simulink model "Rectificador_5_1_2026_optimizado"  (R2024a)
settings: Solver=VariableStepAuto  StartTime=0.0  StopTime=50  RelTol=1e-3
undefined symbols (not defined in the file): D1, Delta, DiscIntNeverNeededParam
libraries: spsSeriesRLCBranchLib x29, spsGroundLib x8, spsabctodq0Lib x4, simulink x4, spsUniversalBridgeLib x3, spsThreePhaseVIMeasurementLib x3, spsRMSLib x2, spsPWMGenerator2LevelLib x2, spsVoltageMeasurementLib x1, spsPower3phInstantaneousLib x1, spsPermanentMagnetSynchronousMachineLib x1, spsThreePhaseSourceLib x1
settings Model: PacingRate=1000  Creator=User  LastModifiedBy=User

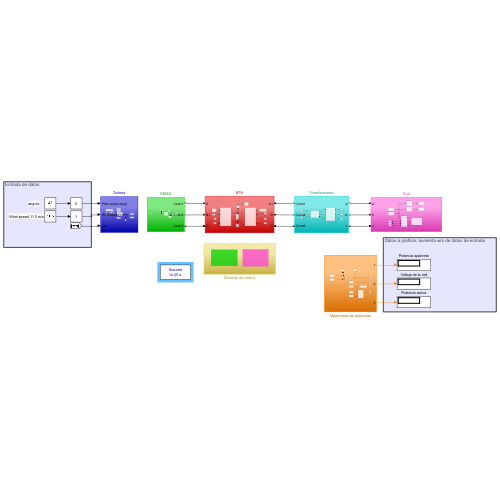
[thumbnail: Simulink's stored preview of the top-level diagram]
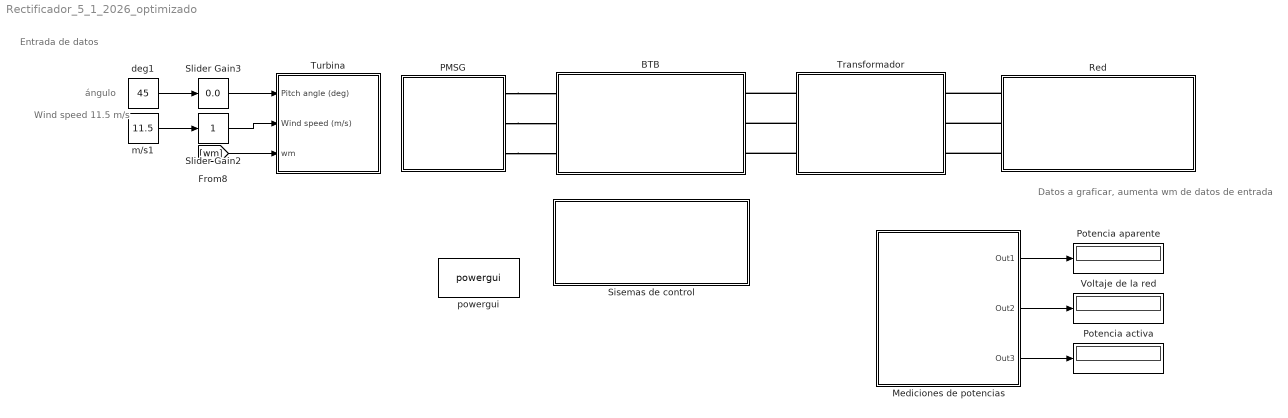
== system Rectificador_5_1_2026_optimizado ==
  note: Datos a graficar, aumenta wm de datos de entrada
  note: Wind speed 11.5 m/s
  note: ángulo
  note: Entrada de datos
  BTB : Subsystem
  Mediciones de potencias : Subsystem
  PMSG : Subsystem
  Potencia activa : Display
  Potencia aparente : Display
  Red : Subsystem
  Sisemas de control : Subsystem
  Slider Gain2 : simulink/Math Operations/Slider Gain  gain=1  low=0.2  high=1.0434782609
  Slider Gain3 : simulink/Math Operations/Slider Gain  gain=0.0  low=0  high=1
  Transformador : Subsystem
  Turbina : Subsystem
  Voltaje de la red : Display
  deg1 : Constant  Value=45  SampleTime=1e-6
  m/s1 : Constant  Value=11.5  SampleTime=1e-6
  powergui : spspowerguiLib/powergui  Priority=1  SimulationMode=Discrete  SampleTime=1e-5  frequency=60  Iterations=50  frequencyindice=0  Pbase=100e6  ErrMax=1e-4  UnitsV=kV  UnitsW=MW  buscounter=0  FunctionMessages=off  echomessages=off  EnableUseOfTLC=off  CurrentSourceSwitches=off  DisableSnubberDevices=off  DisableRonSwitches=off  DisableVfSwitches=off  DisplayEquations=off  AutomaticDiscreteSolvers=off  SolverType=Tustin/Backward Euler (TBE)  Interpol=off  ExternalGateDelay=off  methode=off  Ts=100  x0status=blocks  SPID=on  SwTol=0  HookPort=off  NonlinearTolerance=1e-4  nMaxIteration=100  ContinueOnMaxIteration=off  RestoreLinks=warning  ResistiveCurrentMeasurement=off  Frange=[0:2:500]  Ylog=off  Xlog=on  ShowGrid=off  save=off  variable=ZData  structure=0  ZoomFFT=off  StartTime=0.0  cycles=1  DisplayStyle=1  fundamental=60  FreqAxis=off  MaxFrequency=1000  frequencyindicesteady=1  RmsSteady=1  display=off
  wires:
  Slider Gain3/1 -> Turbina/1(Pitch angle (deg))
  deg1/1 -> Slider Gain3/1
  Slider Gain2/1 -> Turbina/2(Wind speed (m/s))
  m/s1/1 -> Slider Gain2/1
  [wm] -> Turbina/3(wm)
  Mediciones de potencias/1(Out1) -> Potencia aparente/1
  Mediciones de potencias/2(Out2) -> Voltaje de la red/1
  Mediciones de potencias/3(Out3) -> Potencia activa/1
  connections:
  PMSG/LConn1 -- BTB/RConn1
  PMSG/LConn2 -- BTB/RConn2
  PMSG/LConn3 -- BTB/RConn3
  Transformador/RConn1 -- BTB/LConn1
  Transformador/RConn2 -- BTB/LConn2
  Transformador/RConn3 -- BTB/LConn3
  Red/RConn1 -- Transformador/LConn1
  Red/RConn2 -- Transformador/LConn2
  Red/RConn3 -- Transformador/LConn3

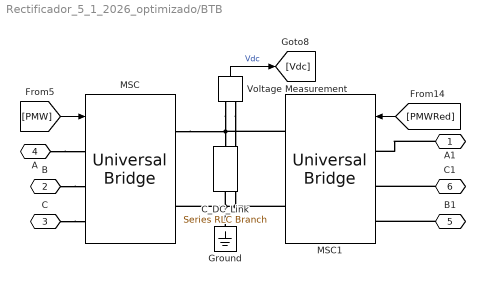
== system Rectificador_5_1_2026_optimizado/BTB ==
  C_DC_Link : spsSeriesRLCBranchLib/Series RLC Branch  LConnTagsString=__new0  RConnTagsString=__new0  BranchType=C  Resistance=1  Inductance=1e-3  SetiL0=off  InitialCurrent=0  Capacitance=5000e-6  Setx0=on  InitialVoltage=0  Measurements=None
  Ground : spsGroundLib/Ground  LConnTagsString=a
  MSC : spsUniversalBridgeLib/Universal Bridge  Arms=3  SnubberResistance=1e5  SnubberCapacitance=inf  Device=IGBT / Diodes  Ron=1e-3  Lon=0  ForwardVoltages=[ 0.8 , 0.8 ]  ForwardVoltage=0  GTOparameters=[ 10e-6 , 20e-6 ]  IGBTparameters=[ 1e-6 , 2e-6 ]  Measurements=None  Measurements_2=None  converterType=Rectifier
  MSC1 : spsUniversalBridgeLib/Universal Bridge  Arms=3  SnubberResistance=1e5  SnubberCapacitance=inf  Device=IGBT / Diodes  Ron=1e-3  Lon=0  ForwardVoltages=[ 0.8 , 0.8 ]  ForwardVoltage=0  GTOparameters=[ 10e-6 , 20e-6 ]  IGBTparameters=[ 1e-6 , 2e-6 ]  Measurements=None  Measurements_2=None  converterType=Rectifier
  Voltage Measurement : spsVoltageMeasurementLib/Voltage Measurement  PhasorSimulation=off  OutputType=Complex  PSBequivalent=0
  A1 : PMIOPort  Side=Left
  B : PMIOPort  Port=2  Side=Left
  C : PMIOPort  Port=3  Side=Left
  A : PMIOPort  Port=4  Side=Right
  B1 : PMIOPort  Port=5  Side=Right
  C1 : PMIOPort  Port=6  Side=Right
  wires:
  Voltage Measurement/1 -> [Vdc]  "Vdc"
  [PMWRed] -> MSC1/1
  [PMW] -> MSC/1
  connections:
  Voltage Measurement/LConn1 -- MSC1/RConn1 -- MSC/RConn1 -- C_DC_Link/LConn1
  A1/RConn1 -- MSC1/LConn1
  Voltage Measurement/LConn2 -- MSC/RConn2 -- Ground/LConn1 -- C_DC_Link/RConn1 -- MSC1/RConn2
  A/RConn1 -- MSC/LConn1
  B/RConn1 -- MSC/LConn2
  C/RConn1 -- MSC/LConn3
  C1/RConn1 -- MSC1/LConn2
  B1/RConn1 -- MSC1/LConn3

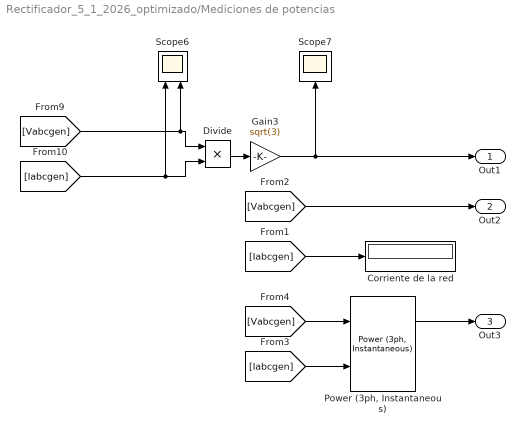
== system Rectificador_5_1_2026_optimizado/Mediciones de potencias ==
  Corriente de la red : Display
  Divide : Product  Inputs=**
  Gain3 : Gain  Gain=sqrt(3)
  "Power (3ph, Instantaneous)" : spsPower3phInstantaneousLib/Power (3ph, Instantaneous)
  Scope6 : Scope  NumInputPorts=2
  Scope7 : Scope
  Out1 : Outport
  Out2 : Outport  Port=2
  Out3 : Outport  Port=3
  wires:
  [Iabcgen] -> Divide/2, Scope6/2
  Gain3/1 -> Out1/1, Scope7/1
  [Iabcgen] -> Corriente de la red/1
  Divide/1 -> Gain3/1
  [Vabcgen] -> Scope6/1, Divide/1
  [Vabcgen] -> Out2/1
  [Vabcgen] -> "Power (3ph, Instantaneous)"/1
  [Iabcgen] -> "Power (3ph, Instantaneous)"/2
  "Power (3ph, Instantaneous)"/1 -> Out3/1

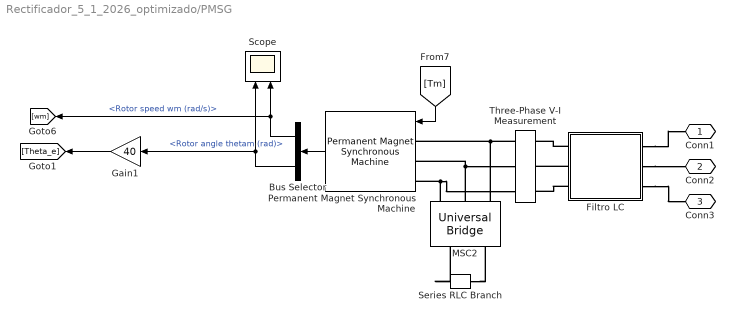
== system Rectificador_5_1_2026_optimizado/PMSG ==
  Bus Selector : BusSelector  OutputSignals=Rotor speed wm (rad/s),Rotor angle thetam (rad)
  Filtro LC : Subsystem
  Gain1 : Gain  Gain=40
  MSC2 : spsUniversalBridgeLib/Universal Bridge  Arms=3  SnubberResistance=1e5  SnubberCapacitance=inf  Device=Diodes  Ron=1e-3  Lon=0  ForwardVoltages=[ 0.8 , 0.8 ]  ForwardVoltage=0  GTOparameters=[ 10e-6 , 20e-6 ]  IGBTparameters=[ 1e-6 , 2e-6 ]  Measurements=None  Measurements_2=None  converterType=Rectifier
  Permanent Magnet Synchronous Machine : spsPermanentMagnetSynchronousMachineLib/Permanent Magnet Synchronous Machine  NbPhases=3  FluxDistribution=Sinusoidal  RotorType=Round  MechanicalLoad=Torque Tm  PresetModel=No  ShowDetailedParameters=on  MeasurementBus=off  Resistance=0.004  Inductance=8.5e-3  dqInductances=[8.5e-3,8.5e-3]  La=0.00175  MachineConstant=Flux linkage established by magnets (V.s)  Flux=5.85787  VoltageCst=42500.0035  TorqueCst=351.4722  Flat=120  Mechanical=[4e+06 1000 40]  PolePairs=4  InitialConditions=[0,0, 0,0]  InitialConditions5ph=[0 0 0 0 0 0]  RefAngle=90 degrees behind phase A axis (modified Park)  IterativeDiscreteModel=Trapezoidal non iterative  TsBlock=1e-06  TsPowergui=0
  Scope : Scope  NumInputPorts=2
  Series RLC Branch : spsSeriesRLCBranchLib/Series RLC Branch  LConnTagsString=__new0  RConnTagsString=__new0  BranchType=R  Resistance=100000  Inductance=1e-3  SetiL0=off  InitialCurrent=0  Capacitance=1e-6  Setx0=off  InitialVoltage=0  Measurements=None
  Three-Phase V-I Measurement : spsThreePhaseVIMeasurementLib/Three-Phase V-I Measurement  VoltageMeasurement=phase-to-ground  SetLabelV=on  LabelV=Vabc_gen  Vpu=off  VpuLL=off  CurrentMeasurement=yes  SetLabelI=on  LabelI=Iabc_gen  Ipu=off  Pbase=100e6  Vbase=500e3  OutputType=Complex  PhasorSimulation=off  PSBequivalent=0
  Conn1 : PMIOPort  Side=Left
  Conn2 : PMIOPort  Port=2  Side=Left
  Conn3 : PMIOPort  Port=3  Side=Left
  wires:
  Bus Selector/2 -> Gain1/1, Scope/2  "<Rotor angle thetam (rad)>"
  Gain1/1 -> [Theta_e]
  [Tm] -> Permanent Magnet Synchronous Machine/1
  Bus Selector/1 -> Scope/1, [wm]  "<Rotor speed wm (rad/s)>"
  Permanent Magnet Synchronous Machine/1 -> Bus Selector/1
  connections:
  Three-Phase V-I Measurement/RConn1 -- Permanent Magnet Synchronous Machine/LConn1 -- MSC2/LConn1
  MSC2/LConn2 -- Permanent Magnet Synchronous Machine/LConn2 -- Three-Phase V-I Measurement/RConn2
  MSC2/LConn3 -- Three-Phase V-I Measurement/RConn3 -- Permanent Magnet Synchronous Machine/LConn3
  Filtro LC/RConn3 -- Three-Phase V-I Measurement/LConn3
  Series RLC Branch/RConn1 -- MSC2/RConn2
  Filtro LC/RConn2 -- Three-Phase V-I Measurement/LConn2
  Series RLC Branch/LConn1 -- MSC2/RConn1
  Filtro LC/RConn1 -- Three-Phase V-I Measurement/LConn1
  Filtro LC/LConn2 -- Conn2/RConn1
  Filtro LC/LConn3 -- Conn3/RConn1
  Filtro LC/LConn1 -- Conn1/RConn1

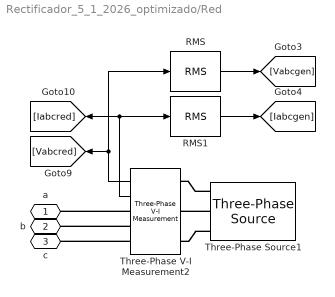
== system Rectificador_5_1_2026_optimizado/Red ==
  RMS : spsRMSLib/RMS  TrueRMS=on  Freq=60  RMSInit=120  Ts=1e-6
  RMS1 : spsRMSLib/RMS  TrueRMS=on  Freq=60  RMSInit=120  Ts=1e-6
  Three-Phase V-I Measurement2 : spsThreePhaseVIMeasurementLib/Three-Phase V-I Measurement  VoltageMeasurement=phase-to-phase  SetLabelV=off  LabelV=Vabc  Vpu=off  VpuLL=off  CurrentMeasurement=yes  SetLabelI=off  LabelI=Iabc  Ipu=off  Pbase=100e6  Vbase=500e3  OutputType=Complex  PhasorSimulation=off  PSBequivalent=0
  Three-Phase Source1 : spsThreePhaseSourceLib/Three-Phase Source  InternalConnection=Yg  VoltagePhases=off  Voltage=34.5e3  PhaseAngle=0  Voltage_phases=[25e3 25e3 25e3]/sqrt(3)  PhaseAngles_phases=[0 -120 +120]  Frequency=60  NonIdealSource=on  SpecifyImpedance=off  Resistance=1e-12  Inductance=1e-12  ShortCircuitLevel=100e6  BaseVoltage=34.5e3  XRratio=7  BusType=swing  Pref=10e3  Qref=0  Prefabc=[10e3, 10e3, 10e3]  Qrefabc=[0, 0, 0]  Qmin=-inf  Qmax=inf
  a : PMIOPort  Side=Right
  b : PMIOPort  Port=2  Side=Right
  c : PMIOPort  Port=3  Side=Right
  wires:
  Three-Phase V-I Measurement2/1 -> [Vabcred], RMS/1
  RMS/1 -> [Vabcgen]
  Three-Phase V-I Measurement2/2 -> [Iabcred], RMS1/1
  RMS1/1 -> [Iabcgen]
  connections:
  Three-Phase Source1/RConn2 -- Three-Phase V-I Measurement2/LConn2
  Three-Phase Source1/RConn1 -- Three-Phase V-I Measurement2/LConn1
  Three-Phase V-I Measurement2/RConn2 -- b/RConn1
  Three-Phase Source1/RConn3 -- Three-Phase V-I Measurement2/LConn3
  Three-Phase V-I Measurement2/RConn3 -- c/RConn1
  Three-Phase V-I Measurement2/RConn1 -- a/RConn1

== system Rectificador_5_1_2026_optimizado/Sisemas de control ==
  Sistema control lado de la red : Subsystem
  Sistema de control lado de PMSG : Subsystem

== system Rectificador_5_1_2026_optimizado/Transformador ==
  Filtro LCL : Subsystem
  Three-Phase Transformer (Two Windings) : spsThreePhaseTransformerTwoWindingsLib/Three-Phase Transformer (Two Windings)  Winding1Connection=Delta (D1)  Winding2Connection=Yg  CoreType=Three single-phase transformers  SetSaturation=off  Hysteresis=off  DataFile='hysteresis'  SetInitialFlux=off  Measurements=None  UNITS=SI  NominalPower=[ 4.4e6 , 60 ]  Winding1=[ 690 , 0.00558 , 1.92e-5]  Winding2=[ 34.5e3 ,1.395 , 0.00048]  Rm=1000  Lm=0.5  L0=0.5  Saturation=[0 0;0.66653 1910.3;277.72 2419.7]  InitialFluxes=[ 0.8 , -0.8 , 0.7 ]  BreakLoop=off  DiscreteSolver=Trapezoidal iterative  DataType=on  TransfoNumber=1
  a : PMIOPort  Side=Left
  b : PMIOPort  Port=2  Side=Left
  c : PMIOPort  Port=3  Side=Left
  Conn1 : PMIOPort  Port=4  Side=Right
  Conn4 : PMIOPort  Port=5  Side=Right
  Conn6 : PMIOPort  Port=6  Side=Right
  connections:
  Filtro LCL/RConn2 -- Conn4/RConn1
  Three-Phase Transformer (Two Windings)/LConn3 -- Filtro LCL/LConn3
  Three-Phase Transformer (Two Windings)/LConn2 -- Filtro LCL/LConn2
  a/RConn1 -- Three-Phase Transformer (Two Windings)/RConn1
  c/RConn1 -- Three-Phase Transformer (Two Windings)/RConn3
  Three-Phase Transformer (Two Windings)/LConn1 -- Filtro LCL/LConn1
  Filtro LCL/RConn1 -- Conn1/RConn1
  b/RConn1 -- Three-Phase Transformer (Two Windings)/RConn2
  Filtro LCL/RConn3 -- Conn6/RConn1

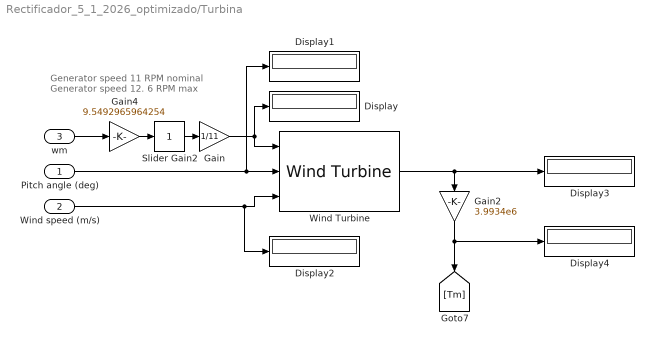
== system Rectificador_5_1_2026_optimizado/Turbina ==
  note: Generator speed 11 RPM nominal
      | Generator speed 12. 6 RPM max
  Pitch angle (deg) : Inport
  Wind speed (m/s) : Inport  Port=2
  wm : Inport  Port=3
  Display{,1..4} (5 alike) : Display
  Gain : Gain  Gain=1/11
  Gain2 : Gain  Gain=3.9934e6
  Gain4 : Gain  Gain=9.5492965964254
  Slider Gain2 : simulink/Math Operations/Slider Gain  gain=1  low=0.2  high=1.145
  Wind Turbine : spsWindTurbineLib/Wind Turbine  Pnom=4.59e6  Pelec_base=4.59e6  wind_base=11.5  P_wind_base=1  speed_nom=1  pitch_angle=0  c1_c6="[0.51763          116          0.4            5           21     0.006795]"  cp_nom=0.48  lambda_nom=8.1
  wires:
  Gain/1 -> Wind Turbine/1, Display/1
  Wind Turbine/1 -> Display3/1, Gain2/1
  Gain4/1 -> Slider Gain2/1
  wm/1 -> Gain4/1
  Gain2/1 -> [Tm], Display4/1
  Pitch angle (deg)/1 -> Display1/1, Wind Turbine/2
  Slider Gain2/1 -> Gain/1
  Wind speed (m/s)/1 -> Wind Turbine/3, Display2/1

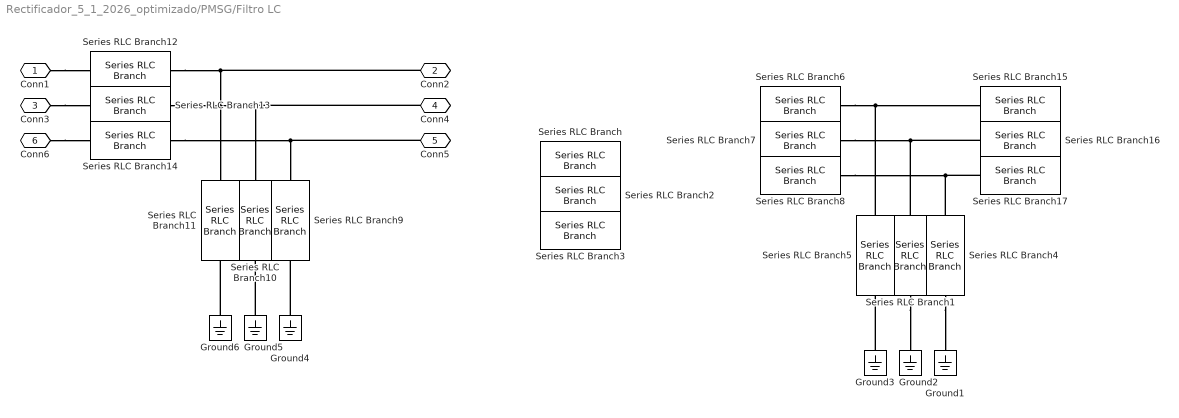
== system Rectificador_5_1_2026_optimizado/PMSG/Filtro LC ==
  Ground{1..6} (6 alike) : spsGroundLib/Ground  LConnTagsString=a
  Series RLC Branch : spsSeriesRLCBranchLib/Series RLC Branch  LConnTagsString=__new0  RConnTagsString=__new0  BranchType=L  Resistance=1  Inductance=8.1685e-06  SetiL0=off  InitialCurrent=0  Capacitance=1e-6  Setx0=off  InitialVoltage=0  Measurements=None
  Series RLC Branch1 : spsSeriesRLCBranchLib/Series RLC Branch  LConnTagsString=__new0  RConnTagsString=__new0  BranchType=RC  Resistance=0  Inductance=1e-3  SetiL0=off  InitialCurrent=0  Capacitance=200e-6  Setx0=off  InitialVoltage=0  Measurements=None
  Series RLC Branch10 : spsSeriesRLCBranchLib/Series RLC Branch  LConnTagsString=__new0  RConnTagsString=__new0  BranchType=RC  Resistance=0.04  Inductance=1e-3  SetiL0=off  InitialCurrent=0  Capacitance=100e-06  Setx0=off  InitialVoltage=0  Measurements=None
  Series RLC Branch11 : spsSeriesRLCBranchLib/Series RLC Branch  LConnTagsString=__new0  RConnTagsString=__new0  BranchType=RC  Resistance=0.04  Inductance=1e-3  SetiL0=off  InitialCurrent=0  Capacitance=100e-06  Setx0=off  InitialVoltage=0  Measurements=None
  Series RLC Branch12 : spsSeriesRLCBranchLib/Series RLC Branch  LConnTagsString=__new0  RConnTagsString=__new0  BranchType=L  Resistance=1  Inductance=50e-04  SetiL0=off  InitialCurrent=0  Capacitance=1e-6  Setx0=off  InitialVoltage=0  Measurements=None
  Series RLC Branch13 : spsSeriesRLCBranchLib/Series RLC Branch  LConnTagsString=__new0  RConnTagsString=__new0  BranchType=L  Resistance=1  Inductance=50e-04  SetiL0=off  InitialCurrent=0  Capacitance=1e-6  Setx0=off  InitialVoltage=0  Measurements=None
  Series RLC Branch14 : spsSeriesRLCBranchLib/Series RLC Branch  LConnTagsString=__new0  RConnTagsString=__new0  BranchType=L  Resistance=1  Inductance=50e-04  SetiL0=off  InitialCurrent=0  Capacitance=1e-6  Setx0=off  InitialVoltage=0  Measurements=None
  Series RLC Branch15 : spsSeriesRLCBranchLib/Series RLC Branch  LConnTagsString=__new0  RConnTagsString=__new0  BranchType=L  Resistance=0  Inductance=0.1e-3  SetiL0=off  InitialCurrent=0  Capacitance=1e-6  Setx0=off  InitialVoltage=0  Measurements=None
  Series RLC Branch16 : spsSeriesRLCBranchLib/Series RLC Branch  LConnTagsString=__new0  RConnTagsString=__new0  BranchType=L  Resistance=0  Inductance=0.1e-3  SetiL0=off  InitialCurrent=0  Capacitance=1e-6  Setx0=off  InitialVoltage=0  Measurements=None
  Series RLC Branch17 : spsSeriesRLCBranchLib/Series RLC Branch  LConnTagsString=__new0  RConnTagsString=__new0  BranchType=L  Resistance=0  Inductance=0.1e-3  SetiL0=off  InitialCurrent=0  Capacitance=1e-6  Setx0=off  InitialVoltage=0  Measurements=None
  Series RLC Branch2 : spsSeriesRLCBranchLib/Series RLC Branch  LConnTagsString=__new0  RConnTagsString=__new0  BranchType=L  Resistance=1  Inductance=8.1685e-06  SetiL0=off  InitialCurrent=0  Capacitance=1e-6  Setx0=off  InitialVoltage=0  Measurements=None
  Series RLC Branch3 : spsSeriesRLCBranchLib/Series RLC Branch  LConnTagsString=__new0  RConnTagsString=__new0  BranchType=L  Resistance=1  Inductance=8.1685e-06  SetiL0=off  InitialCurrent=0  Capacitance=1e-6  Setx0=off  InitialVoltage=0  Measurements=None
  Series RLC Branch4 : spsSeriesRLCBranchLib/Series RLC Branch  LConnTagsString=__new0  RConnTagsString=__new0  BranchType=RC  Resistance=0  Inductance=1e-3  SetiL0=off  InitialCurrent=0  Capacitance=200e-6  Setx0=off  InitialVoltage=0  Measurements=None
  Series RLC Branch5 : spsSeriesRLCBranchLib/Series RLC Branch  LConnTagsString=__new0  RConnTagsString=__new0  BranchType=RC  Resistance=0  Inductance=1e-3  SetiL0=off  InitialCurrent=0  Capacitance=200e-6  Setx0=off  InitialVoltage=0  Measurements=None
  Series RLC Branch6 : spsSeriesRLCBranchLib/Series RLC Branch  LConnTagsString=__new0  RConnTagsString=__new0  BranchType=L  Resistance=0  Inductance=3e-3  SetiL0=off  InitialCurrent=0  Capacitance=1e-6  Setx0=off  InitialVoltage=0  Measurements=None
  Series RLC Branch7 : spsSeriesRLCBranchLib/Series RLC Branch  LConnTagsString=__new0  RConnTagsString=__new0  BranchType=L  Resistance=0  Inductance=3e-3  SetiL0=off  InitialCurrent=0  Capacitance=1e-6  Setx0=off  InitialVoltage=0  Measurements=None
  Series RLC Branch8 : spsSeriesRLCBranchLib/Series RLC Branch  LConnTagsString=__new0  RConnTagsString=__new0  BranchType=L  Resistance=0  Inductance=3e-3  SetiL0=off  InitialCurrent=0  Capacitance=1e-6  Setx0=off  InitialVoltage=0  Measurements=None
  Series RLC Branch9 : spsSeriesRLCBranchLib/Series RLC Branch  LConnTagsString=__new0  RConnTagsString=__new0  BranchType=RC  Resistance=0.04  Inductance=1e-3  SetiL0=off  InitialCurrent=0  Capacitance=100e-06  Setx0=off  InitialVoltage=0  Measurements=None
  Conn1 : PMIOPort  Side=Left
  Conn2 : PMIOPort  Port=2  Side=Right
  Conn3 : PMIOPort  Port=3  Side=Left
  Conn4 : PMIOPort  Port=4  Side=Right
  Conn5 : PMIOPort  Port=5  Side=Right
  Conn6 : PMIOPort  Port=6  Side=Left
  connections:
  Series RLC Branch4/RConn1 -- Ground1/LConn1
  Series RLC Branch1/RConn1 -- Ground2/LConn1
  Ground3/LConn1 -- Series RLC Branch5/RConn1
  Series RLC Branch6/RConn1 -- Series RLC Branch5/LConn1 -- Series RLC Branch15/LConn1
  Series RLC Branch7/RConn1 -- Series RLC Branch1/LConn1 -- Series RLC Branch16/LConn1
  Series RLC Branch8/RConn1 -- Series RLC Branch4/LConn1 -- Series RLC Branch17/LConn1
  Series RLC Branch13/RConn1 -- Conn4/RConn1 -- Series RLC Branch10/LConn1
  Series RLC Branch12/RConn1 -- Conn2/RConn1 -- Series RLC Branch11/LConn1
  Series RLC Branch14/RConn1 -- Conn5/RConn1 -- Series RLC Branch9/LConn1
  Ground6/LConn1 -- Series RLC Branch11/RConn1
  Ground4/LConn1 -- Series RLC Branch9/RConn1
  Ground5/LConn1 -- Series RLC Branch10/RConn1
  Conn1/RConn1 -- Series RLC Branch12/LConn1
  Conn3/RConn1 -- Series RLC Branch13/LConn1
  Conn6/RConn1 -- Series RLC Branch14/LConn1

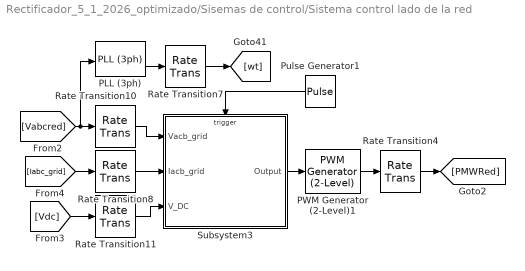
== system Rectificador_5_1_2026_optimizado/Sisemas de control/Sistema control lado de la red ==
  PLL (3ph) : spsPLL3phLib/PLL (3ph)  Fmin=45  Par_Init=[0, 60]  ParK=[180, 3200, 1]  TcD=1e-4  MaxRateChangeFreq=12  FilterCutOffFreq=25  Ts=0  AGC=on
  PWM Generator (2-Level)1 : spsPWMGenerator2LevelLib/PWM Generator (2-Level)  ModulatorType=Three-phase bridge (6 pulses)  ModulatorMode=Unsynchronized  Fc=10000  Pc=90  nF=27  MinMax="[ -1  1 ]"  SamplingTechnique=Natural  ModulatingSignals=off  m=0.8  Freq=60  Phase=0  Ts=1e-6  ShowCarrierOutport=off
  Pulse Generator1 : DiscretePulseGenerator  PulseType=Time based  Period=1e-3  PulseWidth=50
  Rate Transition{4,7..8,10..11} (5 alike) : RateTransition
  Subsystem3 : Subsystem
  wires:
  Rate Transition10/1 -> Subsystem3/1(Vacb_grid)
  [Vabcred] -> PLL (3ph)/1, Rate Transition10/1
  Subsystem3/1(Output) -> PWM Generator (2-Level)1/1
  Pulse Generator1/1 -> Subsystem3/Trigger
  Rate Transition7/1 -> [wt]
  Rate Transition11/1 -> Subsystem3/3(V_DC)
  [Iabc_grid] -> Rate Transition8/1
  [Vdc] -> Rate Transition11/1
  Rate Transition4/1 -> [PMWRed]
  Rate Transition8/1 -> Subsystem3/2(Iacb_grid)
  PLL (3ph)/2 -> Rate Transition7/1
  PWM Generator (2-Level)1/1 -> Rate Transition4/1

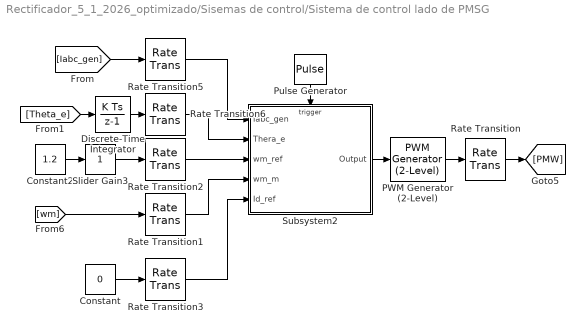
== system Rectificador_5_1_2026_optimizado/Sisemas de control/Sistema de control lado de PMSG ==
  Constant : Constant  Value=0  SampleTime=-1
  Constant2 : Constant  Value=1.2  SampleTime=-1
  Discrete-Time Integrator : DiscreteIntegrator  SampleTime=-1  ICPrevOutput=DiscIntNeverNeededParam  ICPrevScaledInput=DiscIntNeverNeededParam
  PWM Generator (2-Level) : spsPWMGenerator2LevelLib/PWM Generator (2-Level)  ModulatorType=Three-phase bridge (6 pulses)  ModulatorMode=Unsynchronized  Fc=10000  Pc=90  nF=27  MinMax="[ -1  1 ]"  SamplingTechnique=Natural  ModulatingSignals=off  m=0.8  Freq=60  Phase=0  Ts=1e-6  ShowCarrierOutport=off
  Pulse Generator : DiscretePulseGenerator  PulseType=Time based  Period=1e-3  PulseWidth=50
  Rate Transition{,1..3,5..6} (6 alike) : RateTransition
  Slider Gain3 : simulink/Math Operations/Slider Gain  gain=1  low=0.2  high=1.145
  Subsystem2 : Subsystem
  wires:
  PWM Generator (2-Level)/1 -> Rate Transition/1
  Pulse Generator/1 -> Subsystem2/Trigger
  Discrete-Time Integrator/1 -> Rate Transition6/1
  Subsystem2/1(Output) -> PWM Generator (2-Level)/1
  Rate Transition2/1 -> Subsystem2/3(wm_ref)
  Rate Transition5/1 -> Subsystem2/1(Iabc_gen)
  Rate Transition6/1 -> Subsystem2/2(Thera_e)
  [Iabc_gen] -> Rate Transition5/1
  Slider Gain3/1 -> Rate Transition2/1
  Rate Transition/1 -> [PMW]
  [Theta_e] -> Discrete-Time Integrator/1
  Constant/1 -> Rate Transition3/1
  Rate Transition1/1 -> Subsystem2/4(wm_m)
  [wm] -> Rate Transition1/1
  Rate Transition3/1 -> Subsystem2/5(Id_ref)
  Constant2/1 -> Slider Gain3/1

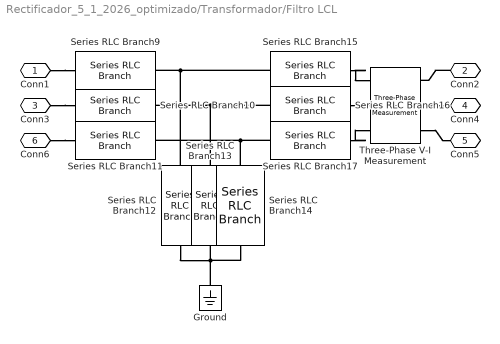
== system Rectificador_5_1_2026_optimizado/Transformador/Filtro LCL ==
  Ground : spsGroundLib/Ground  LConnTagsString=a
  Series RLC Branch10 : spsSeriesRLCBranchLib/Series RLC Branch  LConnTagsString=__new0  RConnTagsString=__new0  BranchType=RL  Resistance=0.07  Inductance=7.2924e-06  SetiL0=off  InitialCurrent=0  Capacitance=1e-6  Setx0=off  InitialVoltage=0  Measurements=None
  Series RLC Branch11 : spsSeriesRLCBranchLib/Series RLC Branch  LConnTagsString=__new0  RConnTagsString=__new0  BranchType=RL  Resistance=0.07  Inductance=7.2924e-06  SetiL0=off  InitialCurrent=0  Capacitance=1e-6  Setx0=off  InitialVoltage=0  Measurements=None
  Series RLC Branch12 : spsSeriesRLCBranchLib/Series RLC Branch  LConnTagsString=__new0  RConnTagsString=__new0  BranchType=RC  Resistance=0.002  Inductance=1e-3  SetiL0=off  InitialCurrent=0  Capacitance=4.3858e-04  Setx0=off  InitialVoltage=0  Measurements=None
  Series RLC Branch13 : spsSeriesRLCBranchLib/Series RLC Branch  LConnTagsString=__new0  RConnTagsString=__new0  BranchType=RC  Resistance=0.002  Inductance=1e-3  SetiL0=off  InitialCurrent=0  Capacitance=4.3858e-04  Setx0=off  InitialVoltage=0  Measurements=None
  Series RLC Branch14 : spsSeriesRLCBranchLib/Series RLC Branch  LConnTagsString=__new0  RConnTagsString=__new0  BranchType=RC  Resistance=0.002  Inductance=1e-3  SetiL0=off  InitialCurrent=0  Capacitance=4.3858e-04  Setx0=off  InitialVoltage=0  Measurements=None
  Series RLC Branch15 : spsSeriesRLCBranchLib/Series RLC Branch  LConnTagsString=__new0  RConnTagsString=__new0  BranchType=L  Resistance=1  Inductance=1.6043e-04  SetiL0=off  InitialCurrent=0  Capacitance=1e-6  Setx0=off  InitialVoltage=0  Measurements=None
  Series RLC Branch16 : spsSeriesRLCBranchLib/Series RLC Branch  LConnTagsString=__new0  RConnTagsString=__new0  BranchType=L  Resistance=1  Inductance=1.6043e-04  SetiL0=off  InitialCurrent=0  Capacitance=1e-6  Setx0=off  InitialVoltage=0  Measurements=None
  Series RLC Branch17 : spsSeriesRLCBranchLib/Series RLC Branch  LConnTagsString=__new0  RConnTagsString=__new0  BranchType=L  Resistance=1  Inductance=1.6043e-04  SetiL0=off  InitialCurrent=0  Capacitance=1e-6  Setx0=off  InitialVoltage=0  Measurements=None
  Series RLC Branch9 : spsSeriesRLCBranchLib/Series RLC Branch  LConnTagsString=__new0  RConnTagsString=__new0  BranchType=RL  Resistance=0.07  Inductance=7.2924e-06  SetiL0=off  InitialCurrent=0  Capacitance=1e-6  Setx0=off  InitialVoltage=0  Measurements=None
  Three-Phase V-I Measurement : spsThreePhaseVIMeasurementLib/Three-Phase V-I Measurement  VoltageMeasurement=no  SetLabelV=off  LabelV=Vabc  Vpu=off  VpuLL=off  CurrentMeasurement=yes  SetLabelI=on  LabelI=Iabc_grid  Ipu=off  Pbase=100e6  Vbase=500e3  OutputType=Complex  PhasorSimulation=off  PSBequivalent=0
  Conn1 : PMIOPort  Side=Left
  Conn2 : PMIOPort  Port=2  Side=Right
  Conn3 : PMIOPort  Port=3  Side=Left
  Conn4 : PMIOPort  Port=4  Side=Right
  Conn5 : PMIOPort  Port=5  Side=Right
  Conn6 : PMIOPort  Port=6  Side=Left
  connections:
  Series RLC Branch17/LConn1 -- Series RLC Branch14/LConn1 -- Series RLC Branch11/RConn1
  Series RLC Branch12/RConn1 -- Ground/LConn1 -- Series RLC Branch14/RConn1 -- Series RLC Branch13/RConn1
  Series RLC Branch15/LConn1 -- Series RLC Branch12/LConn1 -- Series RLC Branch9/RConn1
  Series RLC Branch16/LConn1 -- Series RLC Branch13/LConn1 -- Series RLC Branch10/RConn1
  Conn1/RConn1 -- Series RLC Branch9/LConn1
  Conn3/RConn1 -- Series RLC Branch10/LConn1
  Conn6/RConn1 -- Series RLC Branch11/LConn1
  Series RLC Branch15/RConn1 -- Three-Phase V-I Measurement/LConn1
  Series RLC Branch16/RConn1 -- Three-Phase V-I Measurement/LConn2
  Series RLC Branch17/RConn1 -- Three-Phase V-I Measurement/LConn3
  Three-Phase V-I Measurement/RConn2 -- Conn4/RConn1
  Conn2/RConn1 -- Three-Phase V-I Measurement/RConn1
  Three-Phase V-I Measurement/RConn3 -- Conn5/RConn1

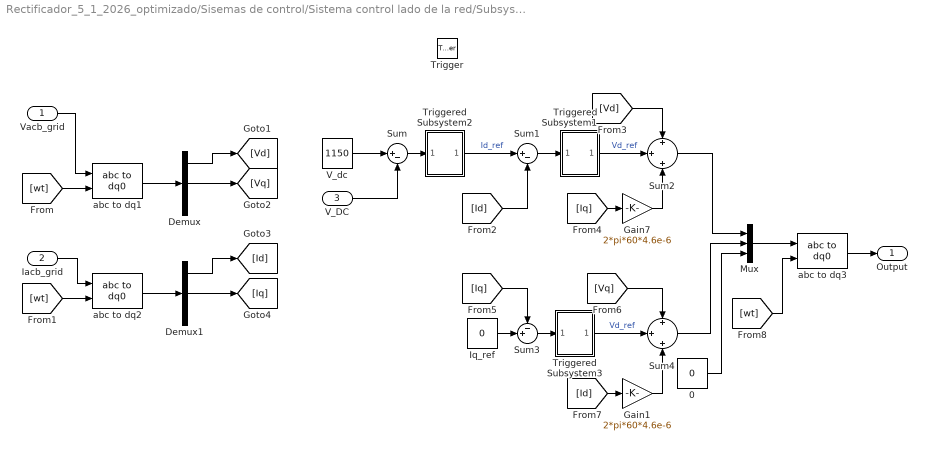
== system Rectificador_5_1_2026_optimizado/Sisemas de control/Sistema control lado de la red/Subsystem3 ==
  Vacb_grid : Inport
  Iacb_grid : Inport  Port=2
  V_DC : Inport  Port=3
  Trigger : TriggerPort  VariantControl=(inherit)
  0 : Constant  Value=0  SampleTime=-1
  Demux : Demux  Outputs=3
  Demux1 : Demux  Outputs=3
  Gain1 : Gain  Gain=2*pi*60*4.6e-6
  Gain7 : Gain  Gain=2*pi*60*4.6e-6
  Iq_ref : Constant  Value=0  SampleTime=-1
  Mux : Mux  Inputs=3
  Sum : Sum  Inputs=|+-
  Sum1 : Sum  Inputs=|+-
  Sum2 : Sum  Inputs=+|+|+
  Sum3 : Sum  Inputs=-+|
  Sum4 : Sum  Inputs=+|+|+
  Triggered Subsystem1 : Subsystem  TreatAsAtomicUnit=on
  Triggered Subsystem2 : Subsystem  TreatAsAtomicUnit=on
  Triggered Subsystem3 : Subsystem  TreatAsAtomicUnit=on
  V_dc : Constant  Value=1150  SampleTime=-1
  abc to dq1 : spsabctodq0Lib/abc to dq0  Alignment=90 degrees behind phase A axis
  abc to dq2 : spsabctodq0Lib/abc to dq0  Alignment=90 degrees behind phase A axis
  abc to dq3 : spsabctodq0Lib/abc to dq0  Alignment=90 degrees behind phase A axis
  Output : Outport
  wires:
  [wt] -> abc to dq1/2
  abc to dq1/1 -> Demux/1
  Demux/1 -> [Vd]
  Demux/2 -> [Vq]
  [wt] -> abc to dq2/2
  Iacb_grid/1 -> abc to dq2/1
  abc to dq2/1 -> Demux1/1
  Demux1/2 -> [Iq]
  Demux1/1 -> [Id]
  V_dc/1 -> Sum/1
  V_DC/1 -> Sum/2
  Sum/1 -> Triggered Subsystem2/1(In1)
  Vacb_grid/1 -> abc to dq1/1
  Triggered Subsystem2/1(Out1) -> Sum1/1  "Id_ref"
  [Id] -> Sum1/2
  Sum1/1 -> Triggered Subsystem1/1(In1)
  Triggered Subsystem1/1(Out1) -> Sum2/2  "Vd_ref"
  [Vd] -> Sum2/1
  [Iq] -> Gain7/1
  Gain7/1 -> Sum2/3
  Iq_ref/1 -> Sum3/2
  [Iq] -> Sum3/1
  Sum3/1 -> Triggered Subsystem3/1(In1)
  Triggered Subsystem3/1(Out1) -> Sum4/2  "Vd_ref"
  [Vq] -> Sum4/1
  [Id] -> Gain1/1
  Gain1/1 -> Sum4/3
  Sum2/1 -> Mux/1
  Sum4/1 -> Mux/2
  0/1 -> Mux/3
  Mux/1 -> abc to dq3/1
  [wt] -> abc to dq3/2
  abc to dq3/1 -> Output/1

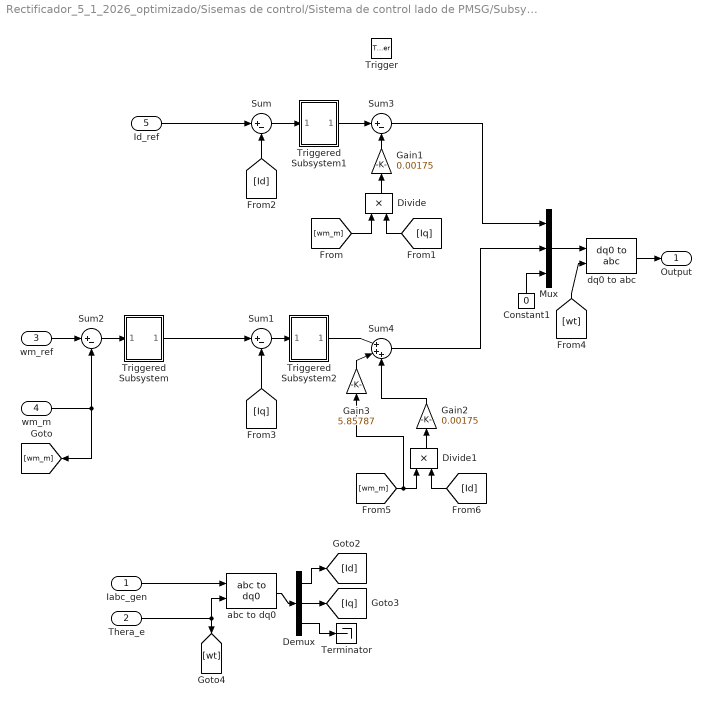
== system Rectificador_5_1_2026_optimizado/Sisemas de control/Sistema de control lado de PMSG/Subsystem2 ==
  Iabc_gen : Inport
  Thera_e : Inport  Port=2
  wm_ref : Inport  Port=3
  wm_m : Inport  Port=4
  Id_ref : Inport  Port=5
  Trigger : TriggerPort  VariantControl=(inherit)
  Constant1 : Constant  Value=0
  Demux : Demux  Outputs=3
  Divide : Product  Inputs=**
  Divide1 : Product  Inputs=**
  Gain1 : Gain  Gain=0.00175
  Gain2 : Gain  Gain=0.00175
  Gain3 : Gain  Gain=5.85787
  Mux : Mux  Inputs=3
  Sum{,1..3} (4 alike) : Sum  Inputs=|+-
  Sum4 : Sum  Inputs=|+++
  Terminator : Terminator
  Triggered Subsystem : Subsystem  TreatAsAtomicUnit=on
  Triggered Subsystem1 : Subsystem  TreatAsAtomicUnit=on
  Triggered Subsystem2 : Subsystem  TreatAsAtomicUnit=on
  abc to dq0 : spsabctodq0Lib/abc to dq0  Alignment=90 degrees behind phase A axis
  dq0 to abc : spsdq0toabcLib/dq0 to abc  Alignment=90 degrees behind phase A axis
  Output : Outport
  wires:
  [Id] -> Sum/2
  Sum/1 -> Triggered Subsystem1/1(In1)
  Sum2/1 -> Triggered Subsystem/1(In1)
  wm_ref/1 -> Sum2/1
  Demux/2 -> [Iq]
  Demux/1 -> [Id]
  [wt] -> dq0 to abc/2
  Sum1/1 -> Triggered Subsystem2/1(In1)
  [Iq] -> Sum1/2
  Mux/1 -> dq0 to abc/1
  abc to dq0/1 -> Demux/1
  Thera_e/1 -> [wt], abc to dq0/2
  Demux/3 -> Terminator/1
  Constant1/1 -> Mux/3
  dq0 to abc/1 -> Output/1
  Iabc_gen/1 -> abc to dq0/1
  wm_m/1 -> Sum2/2, [wm_m]
  Id_ref/1 -> Sum/1
  Triggered Subsystem1/1(Out1) -> Sum3/1
  Sum3/1 -> Mux/1
  Gain1/1 -> Sum3/2
  Divide/1 -> Gain1/1
  [Iq] -> Divide/2
  [wm_m] -> Divide/1
  Triggered Subsystem2/1(Out1) -> Sum4/1
  Gain2/1 -> Sum4/3
  Divide1/1 -> Gain2/1
  [wm_m] -> Gain3/1, Divide1/1
  [Id] -> Divide1/2
  Gain3/1 -> Sum4/2
  Sum4/1 -> Mux/2
  Triggered Subsystem/1(Out1) -> Sum1/1

== system Rectificador_5_1_2026_optimizado/Sisemas de control/Sistema control lado de la red/Subsystem3/Triggered Subsystem1 ==
  In1 : Inport
  Add : Sum
  Discrete-Time Integrator : DiscreteIntegrator  SampleTime=-1  IgnoreLimit=on  ICPrevOutput=DiscIntNeverNeededParam  ICPrevScaledInput=DiscIntNeverNeededParam
  Gain : Gain  Gain=0.0602
  Gain1 : Gain  Gain=5000
  Saturation : Saturate  UpperLimit=1150  LowerLimit=-1150
  Out1 : Outport
  wires:
  Gain1/1 -> Discrete-Time Integrator/1
  Discrete-Time Integrator/1 -> Add/2
  Gain/1 -> Add/1
  In1/1 -> Gain1/1, Gain/1
  Add/1 -> Out1/1

== system Rectificador_5_1_2026_optimizado/Sisemas de control/Sistema control lado de la red/Subsystem3/Triggered Subsystem2 ==
  In1 : Inport
  Add : Sum
  Discrete-Time Integrator : DiscreteIntegrator  SampleTime=-1  IgnoreLimit=on  ICPrevOutput=DiscIntNeverNeededParam  ICPrevScaledInput=DiscIntNeverNeededParam
  Gain : Gain  Gain=379.5
  Gain1 : Gain  Gain=0.031
  Saturation : Saturate  UpperLimit=1150  LowerLimit=-1150
  Out1 : Outport
  wires:
  Gain1/1 -> Discrete-Time Integrator/1
  Discrete-Time Integrator/1 -> Add/2
  Gain/1 -> Add/1
  In1/1 -> Gain1/1, Gain/1
  Add/1 -> Saturation/1
  Saturation/1 -> Out1/1

== system Rectificador_5_1_2026_optimizado/Sisemas de control/Sistema control lado de la red/Subsystem3/Triggered Subsystem3 ==
  In1 : Inport
  Add : Sum
  Discrete-Time Integrator : DiscreteIntegrator  SampleTime=-1  IgnoreLimit=on  ICPrevOutput=DiscIntNeverNeededParam  ICPrevScaledInput=DiscIntNeverNeededParam
  Gain : Gain  Gain=0.0602
  Gain1 : Gain  Gain=5000
  Saturation : Saturate  UpperLimit=1150  LowerLimit=-1150
  Out1 : Outport
  wires:
  Gain1/1 -> Discrete-Time Integrator/1
  Discrete-Time Integrator/1 -> Add/2
  Gain/1 -> Add/1
  In1/1 -> Gain1/1, Gain/1
  Add/1 -> Out1/1

== system Rectificador_5_1_2026_optimizado/Sisemas de control/Sistema de control lado de PMSG/Subsystem2/Triggered Subsystem ==
  In1 : Inport
  Add : Sum
  Discrete-Time Integrator : DiscreteIntegrator  SampleTime=-1  IgnoreLimit=on  ICPrevOutput=DiscIntNeverNeededParam  ICPrevScaledInput=DiscIntNeverNeededParam
  Gain : Gain
  Gain1 : Gain  Gain=50
  Saturation : Saturate  UpperLimit=4.5e6  LowerLimit=-4.5e6
  Out1 : Outport
  wires:
  Gain1/1 -> Discrete-Time Integrator/1
  Discrete-Time Integrator/1 -> Add/2
  Gain/1 -> Add/1
  In1/1 -> Gain1/1, Gain/1
  Add/1 -> Out1/1

== system Rectificador_5_1_2026_optimizado/Sisemas de control/Sistema de control lado de PMSG/Subsystem2/Triggered Subsystem1 ==
  In1 : Inport
  Add : Sum
  Discrete-Time Integrator : DiscreteIntegrator  SampleTime=-1  IgnoreLimit=on  ICPrevOutput=DiscIntNeverNeededParam  ICPrevScaledInput=DiscIntNeverNeededParam
  Gain : Gain  Gain=0.0602
  Gain1 : Gain  Gain=0.031
  Saturation : Saturate  UpperLimit=1150  LowerLimit=-1150
  Out1 : Outport
  wires:
  Gain1/1 -> Discrete-Time Integrator/1
  Discrete-Time Integrator/1 -> Add/2
  Gain/1 -> Add/1
  In1/1 -> Gain1/1, Gain/1
  Add/1 -> Out1/1

== system Rectificador_5_1_2026_optimizado/Sisemas de control/Sistema de control lado de PMSG/Subsystem2/Triggered Subsystem2 ==
  In1 : Inport
  Add : Sum
  Discrete-Time Integrator : DiscreteIntegrator  SampleTime=-1  IgnoreLimit=on  ICPrevOutput=DiscIntNeverNeededParam  ICPrevScaledInput=DiscIntNeverNeededParam
  Gain : Gain  Gain=0.0602
  Gain1 : Gain  Gain=0.031
  Saturation : Saturate  UpperLimit=1150  LowerLimit=-1150
  Out1 : Outport
  wires:
  Gain1/1 -> Discrete-Time Integrator/1
  Discrete-Time Integrator/1 -> Add/2
  Gain/1 -> Add/1
  In1/1 -> Gain1/1, Gain/1
  Add/1 -> Out1/1
